simulink model "PMDCM_PID_2"  (R2022b)
settings: Solver=VariableStepAuto  StartTime=0.0  StopTime=10  RelTol=1e-3
values from neighbouring files (symbols this model uses):
  Bm = 0.00236    [parametros.m]
  Jm = 0.0001    [parametros.m]
  Kt = 0.21469    [parametros.m]
  La = 7    [parametros.m]
  Ra = 1.5    [parametros.m]
  Tl = 0.40825    [parametros.m]
undefined symbols (not defined in the file or in its folder): sigbuilder_block
libraries: fuzblock x3, dspsrcs4 x1
settings Model: Creator=jorge  LastModifiedBy=aurel
settings ModelReferenceCC: EnableRefExpFcnMdlSchedulingChecks=on

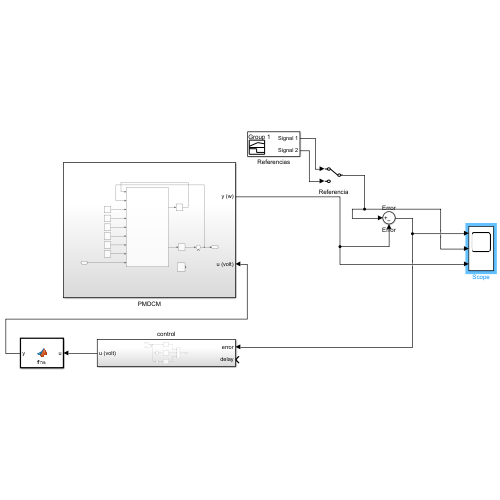
[thumbnail: Simulink's stored preview of the top-level diagram]
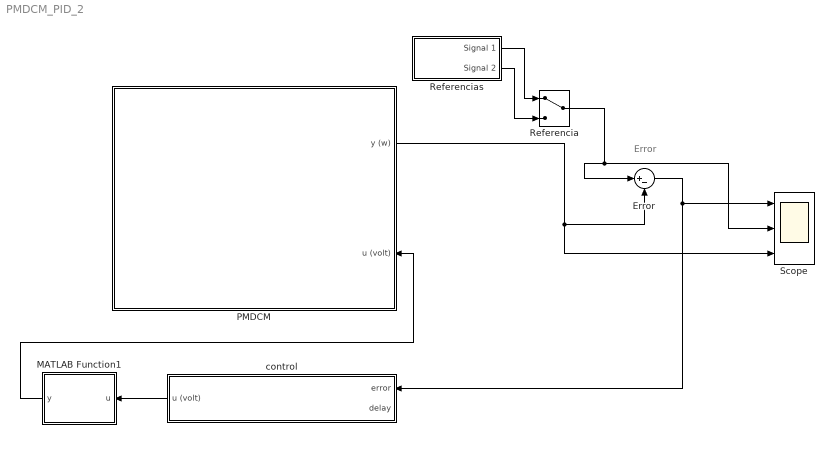
== system PMDCM_PID_2 ==
  note: Error
  Error : Sum  Inputs=|+-
  MATLAB Function1 : MATLAB Function  TreatAsAtomicUnit=on
  PMDCM : Subsystem
      settings: PortSchema="{\"entries\":[{\"content\":{\"sides\":[{\"content\":{\"connectorIds\":[]},\"type\":\"ConnectorPlacement.EquallySpacedRectSide\",\"uuid\":\"65c5596c-c2a0-4a0a-bb90-73b3e0a1ad97\"},{\"content\":{\"connectorIds\":[\"Out1\",\"In1\"],\"side\":\"RIGHT\"},\"type\":\"ConnectorPlacement.EquallySpacedRectSide\",\"uuid\":\"b3efeaed-d3f4-43dc-906b-ae839215104c\"},{\"content\":{\"connectorIds\":[],\"side\":\"TOP\"},\"type\":\"ConnectorPlacement.EquallySpacedRectSide\",\"uuid\":\"106f6a68-3059-4c46-ab15-ef0874f6e17c\"}]},\"type\":\"ConnectorPlacement.EquallySpacedConnector\",\"uuid\":\"214eb961-c195-4fec-8bae-92006976c160\"}],\"packageUris\":[\"http://schema.mathworks.com/mf0/Connector/R2020b\"],\"version\":\"1.0\"}"
  Referencia : ManualSwitch
  Referencias : Subsystem  Tag=STV Subsys  LoadFcn=sigbuilder_block('load');  StartFcn=sigbuilder_block('start');  StopFcn=sigbuilder_block('stop');  ClipboardFcn=sigbuilder_block('clipboard');  mask(Sigbuilder block){tuvar=[0:10]}
      mask help: Simulink:masks:SigbuilderBlock_MD
      mask init:
      | if ~strcmp(get_param(bdroot(gcbh),'SimulationStatus'),'stopped') tuvar = sigbuilder_block('maskInit'); end
      settings: CopyFcn=sigbuilder_block('copy');  DeleteFcn=sigbuilder_block('delete');  ModelCloseFcn=sigbuilder_block('modelClose');  PreSaveFcn=sigbuilder_block('preSave');  PauseFcn=sigbuilder_block('pause');  ContinueFcn=sigbuilder_block('continue');  NameChangeFcn=sigbuilder_block('namechange');  OpenFcn=sigbuilder_block('open',[411 128.5 543.5 351.5 ]);  CloseFcn=sigbuilder_block('close');
      mask Display: plot(0, 0, 100, 100,[2, 2, 32, 32, 2], [68, 8, 8, 68, 68],[32, 2], [38, 38], [32, 19, 2],[53, 60, 44], [32, 17, 17, 2],[16, 16, 31, 31]);txt = getActiveGroup(gcbh);text(2, 100, txt,'verticalAlignment', 'top');
  Scope : Scope  NumInputPorts=3
  control : Subsystem
  wires:
  Error/1 -> control/1(error), Scope/1
  PMDCM/1(y (w)) -> Scope/3, Error/2
  Referencias/1(Signal 1) -> Referencia/1
  Referencias/2(Signal 2) -> Referencia/2
  control/1(u (volt)) -> MATLAB Function1/1(u)
  Referencia/1 -> Error/1, Scope/2
  MATLAB Function1/1(y) -> PMDCM/1(u (volt))

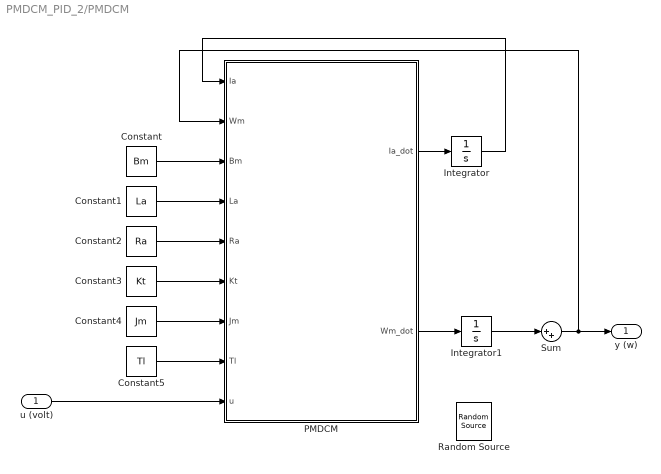
== system PMDCM_PID_2/PMDCM ==
  u (volt) : Inport
  Constant : Constant  Value=Bm
  Constant1 : Constant  Value=La
  Constant2 : Constant  Value=Ra
  Constant3 : Constant  Value=Kt
  Constant4 : Constant  Value=Jm
  Constant5 : Constant  Value=Tl
  Integrator : Integrator
  Integrator1 : Integrator
  PMDCM : MATLAB Function  TreatAsAtomicUnit=on
  Random Source : dspsrcs4/Random Source  SrcType=Uniform  NormMethod=Ziggurat  CltLength=12  MinVal=0  MaxVal=50  MeanVal=0  VarVal=1  RepMode=Not repeatable  rawSeed=1  IsInherit=off  SampMode=Discrete  SampTime=1  SampFrame=1  DataType=Double  OutComplex=Real  OutputFrames=off
  Sum : Sum  Inputs=|++
  y (w) : Outport
  wires:
  PMDCM/2(Wm_dot) -> Integrator1/1
  Integrator/1 -> PMDCM/1(Ia)
  Constant2/1 -> PMDCM/5(Ra)
  Constant5/1 -> PMDCM/8(Tl)
  PMDCM/1(Ia_dot) -> Integrator/1
  Constant/1 -> PMDCM/3(Bm)
  Constant1/1 -> PMDCM/4(La)
  Constant4/1 -> PMDCM/7(Jm)
  Constant3/1 -> PMDCM/6(Kt)
  u (volt)/1 -> PMDCM/9(u)
  Integrator1/1 -> Sum/1
  Sum/1 -> PMDCM/2(Wm), y (w)/1

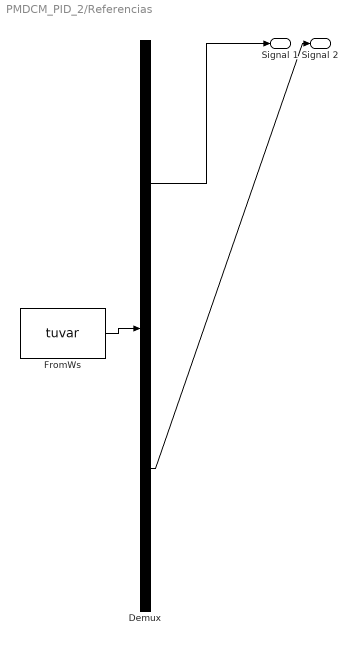
== system PMDCM_PID_2/Referencias ==
  Demux : Demux  Tag=STV Demux  Outputs=2
      settings: DisplayOption=none
  FromWs : FromWorkspace  Tag=STV FromWs  VariableName=tuvar
      SigBuilderData=|
      | common.afterFinalStr = 'Extrapolate'
      | common.sampleTime = 0
      | dataSet.timeRange = [0 10]
      | dataSet.name = 'Group 1'
      | sbobj.Groups.Name = 'Group 1'
      | sbobj.Groups.Signals(1).Name = 'Signal 1'
      | sbobj.Groups.Signals(1).XData = [0 0.001001001001 0.002002002002 0.003003003003 0.004004004004 0.00500500500501 0.00600600600601 0.00700700700701 0.00800800800801 0.00900900900901 0.01001001001 0.011011011011 ... (9991 elements, 1x9991)]
      | sbobj.Groups.Signals(1).YData = [0 0.125788666321 0.251572356775 0.377346095689 0.503104907788 0.628843818382 0.754557853574 0.880242040448 1.00589140727 1.13150098368 1.25706580089 1.3825808919 ... (9991 elements, 1x9991)]
      | sbobj.Groups.Signals(2).Name = 'Signal 2'
      | sbobj.Groups.Signals(2).XData = [0 1 1 2 2 3 3 4 4 5 5 6 6 7 7 8 8 9 9 10]
      | sbobj.Groups.Signals(2).YData = [-20 20 -20 20 -20 20 -20 20 -20 20 -20 20 -20 20 -20 20 -20 20 -20 20]
  Signal 1 : Outport  Tag=STV Outport
  Signal 2 : Outport  Tag=STV Outport  Port=2
  wires:
  Demux/1 -> Signal 1/1
  FromWs/1 -> Demux/1
  Demux/2 -> Signal 2/1

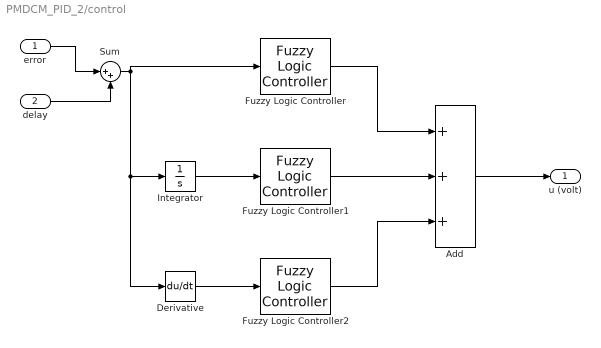
== system PMDCM_PID_2/control ==
  error : Inport
  delay : Inport  Port=2
  Add : Sum  Inputs=+++
  Derivative : Derivative
  Fuzzy Logic Controller : fuzblock/Fuzzy Logic  Controller  FIS='Control_difuso.fis'  OutputSampleNumber=101  DataType=double  FuzzifiedInputs=off  RuleFiringStrengths=off  RuleOutputs=off  AggregatedOutputs=off  SimulateUsing=Interpreted execution  OutOfRangeInputValueMessage=warning  NoRuleFiredMessage=warning  EmptyOutputFuzzySetMessage=warning
  Fuzzy Logic Controller1 : fuzblock/Fuzzy Logic  Controller  FIS='Control_difuso.fis'  OutputSampleNumber=101  DataType=double  FuzzifiedInputs=off  RuleFiringStrengths=off  RuleOutputs=off  AggregatedOutputs=off  SimulateUsing=Interpreted execution  OutOfRangeInputValueMessage=warning  NoRuleFiredMessage=warning  EmptyOutputFuzzySetMessage=warning
  Fuzzy Logic Controller2 : fuzblock/Fuzzy Logic  Controller  FIS='Control_difuso.fis'  OutputSampleNumber=101  DataType=double  FuzzifiedInputs=off  RuleFiringStrengths=off  RuleOutputs=off  AggregatedOutputs=off  SimulateUsing=Interpreted execution  OutOfRangeInputValueMessage=warning  NoRuleFiredMessage=warning  EmptyOutputFuzzySetMessage=warning
  Integrator : Integrator
  Sum : Sum  Inputs=|++
  u (volt) : Outport
  wires:
  Add/1 -> u (volt)/1
  Sum/1 -> Derivative/1, Integrator/1, Fuzzy Logic Controller/1
  Fuzzy Logic Controller/1 -> Add/1
  error/1 -> Sum/1
  delay/1 -> Sum/2
  Integrator/1 -> Fuzzy Logic Controller1/1
  Derivative/1 -> Fuzzy Logic Controller2/1
  Fuzzy Logic Controller1/1 -> Add/2
  Fuzzy Logic Controller2/1 -> Add/3

== matlab function PMDCM_PID_2/PMDCM/PMDCM ==
  data: Ia input; Wm input; Bm input; La input; Ra input; Kt input; Jm input; Tl input; u input; Ia_dot output; Wm_dot output
function [Ia_dot,Wm_dot] = fcn(Ia, Wm, Bm, La, Ra, Kt, Jm, Tl, u)

    Ia_dot = -(Ra/La)*Ia - (Kt/La)*Wm + (1/La)*u;
    Wm_dot = (Kt/Jm)*Ia - (Bm/Jm)*Wm - (1/Jm)*Tl;

end

== matlab function PMDCM_PID_2/MATLAB Function1 ==
  data: u input; y output
function y = fcn(u)
    if u > 15
        y = 15;
    elseif u < -15
        y = -15;
    else
        y = u;
    end
